simulink model "MPC_WoodBerry_2017a"  (R2017a)
settings: Solver=ode3  SolverName=FixedStepAuto  StartTime=0  StopTime=200  FixedStep=Ts  RelTol=1e-3
values from neighbouring files (symbols this model uses):
  L = Tuning_Parameters.scale.L    [Shell3x3.m]    (also in Shell7x5.m; WoodBerry.m; fpso.m; fpso_tuning.m)
  Ru = Tuning_Parameters.scale.Ru    [Shell3x3.m]    (also in Shell7x5.m; WoodBerry.m; fpso.m; fpso1.m = R(1:ny,1:ny))
  Rv = Tuning_Parameters.scale.Rv    [Shell3x3.m]    (also in Shell7x5.m; WoodBerry.m; fpso.m; fpso1.m = R(ny+1:end,ny+1:end))
libraries: cstblocks x2, mpclib x1
settings Model: Creator=Sergio Castaño  LastModifiedBy=Sergio
settings DataIOCC: LimitDataPoints=on
settings OptimizationCC: DefaultParameterBehavior=Inlined  UseFloatMulNetSlope=on  InlineInvariantSignals=on  EnhancedBackFolding=on  PassReuseOutputArgsAs=Individual arguments  EfficientFloat2IntCast=on  LifeSpan=inf
settings DebuggingCC: ParameterTunabilityLossMsg=error  AllowSymbolicDim=off  SFUnexpectedBacktrackingDiag=warning  SFNoUnconditionalDefaultTransitionDiag=warning  SFExecutionAtInitializationDiag=none
settings HardwareCC: ProdBitPerSizeT=32  ProdBitPerPtrDiffT=32  ProdWordSize=32  ProdHWDeviceType=Specified
settings ModelReferenceCC: UpdateModelReferenceTargets=AssumeUpToDate  CheckModelReferenceTargetMessage=none  EnableParallelModelReferenceBuilds=on  PropagateSignalLabelsOutOfModel=off
settings SFSimCC: MATLABDynamicMemAlloc=off
settings RTWCC: SystemTargetFile=ert.tlc  TemplateMakefile=ert_default_tmf  Description=Embedded Coder  GenerateReport=on  IncludeHyperlinkInReport=on  LaunchReport=on  GenerateTraceInfo=on  GenerateTraceReport=on  GenerateTraceReportSl=on  GenerateTraceReportSf=on  GenerateTraceReportEml=on
settings CodeAppCC: ForceParamTrailComments=on  IgnoreCustomStorageClasses=off  OperatorAnnotations=on  SimulinkDataObjDesc=on  SFDataObjDesc=on  InsertBlockDesc=on
settings ERTTargetCC: GenerateSampleERTMain=on  SupportContinuousTime=on  InlinedParameterPlacement=NonHierarchical  ERTCustomFileTemplate=example_file_process.tlc
settings ConfigComp: CovMetricSettings=dw  CovSaveCumulativeToWorkspaceVar=on  CovSaveSingleToWorkspaceVar=on  CovExternalEMLEnable=off

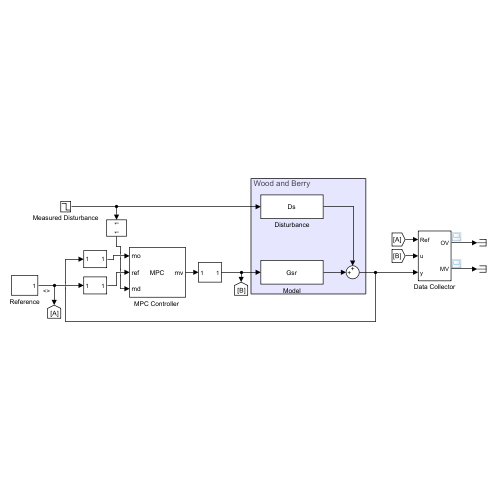
[thumbnail: Simulink's stored preview of the top-level diagram]
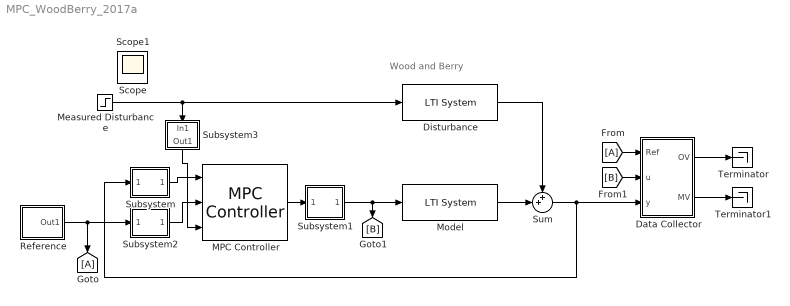
== system MPC_WoodBerry_2017a ==
  note: Wood and Berry
  Data Collector : Subsystem
  Disturbance : cstblocks/LTI System  sys=Ds  IC=[]
  "MPC Controller " : mpclib/MPC Controller  SCDEnableBlockLinearizationSpecification=on  mpcobj=mpc_toolbox  is_multiple=0  enable_value=0  return_u0=off  updateMPCinCallerWorkspace=on  md_inport=on  mv_inport=off  uref_inport=off  cost_outport=off  return_sequence=off  return_qpstatus=off  return_xseq=off  return_state=off  return_ovseq=off  state_inport=off  umin_inport=off  umax_inport=off  ymin_inport=off  ymax_inport=off  cc_inport=off  ywt_inport=off  uwt_inport=off  duwt_inport=off  rhoeps_inport=off  pm_inport=off  MaximumP=10  HorizonChoice=FixedHorizon  n_ts=1  n_p=32  n_mv=2  n_md=1  n_ud=0  n_mo=2  n_uo=0  BlockDataType=double  SampleTimeInherited=off  switch_inport=off
  Measured Disturbance : Step  Time=140  After=-0.25  SampleTime=0
  Model : cstblocks/LTI System  sys=Gsr  IC=[]
  Reference : Subsystem
  Subsystem : Subsystem
  Subsystem1 : Subsystem
  Subsystem2 : Subsystem
  Subsystem3 : Subsystem
  Sum : Sum  Inputs=++|
  Terminator : Terminator
  Terminator1 : Terminator
  Scope : Scope
  Scope1 : Scope
  wires:
  "MPC Controller "/1 -> Subsystem1/1(In1)
  Model/1 -> Sum/2
  Sum/1 -> Data Collector/3(y), Subsystem/1(In1)
  Subsystem/1(Out1) -> "MPC Controller "/1
  Subsystem2/1(Out1) -> "MPC Controller "/2
  Subsystem1/1(Out1) -> [B], Model/1
  Reference/1(Out1) -> [A], Subsystem2/1(In1)
  Measured Disturbance/1 -> Subsystem3/1(In1), Disturbance/1
  [A] -> Data Collector/1(Ref)
  [B] -> Data Collector/2(u)
  Data Collector/1(OV) -> Terminator/1
  Data Collector/2(MV) -> Terminator1/1
  Disturbance/1 -> Sum/1
  Subsystem3/1(Out1) -> "MPC Controller "/3

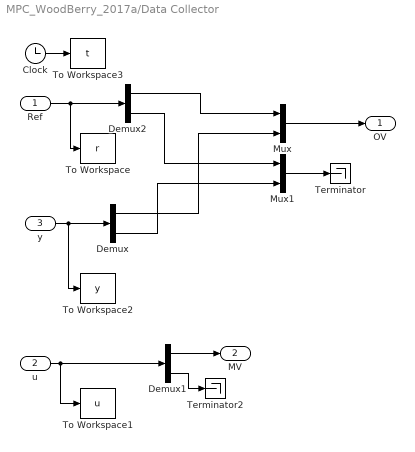
== system MPC_WoodBerry_2017a/Data Collector ==
  Ref : Inport
  u : Inport  Port=2
  y : Inport  Port=3
  Clock : Clock
  Demux : Demux  Outputs=2
  Demux1 : Demux  Outputs=2
  Demux2 : Demux  Outputs=2
  Mux : Mux  Inputs=2
  Mux1 : Mux  Inputs=2
  Terminator : Terminator
  Terminator2 : Terminator
  To Workspace : ToWorkspace  VariableName=r  SampleTime=-1
  To Workspace1 : ToWorkspace  VariableName=u  SampleTime=-1
  To Workspace2 : ToWorkspace  VariableName=y  SampleTime=-1
  To Workspace3 : ToWorkspace  VariableName=t  SampleTime=-1
  OV : Outport
  MV : Outport  Port=2
  wires:
  y/1 -> To Workspace2/1, Demux/1
  u/1 -> Demux1/1, To Workspace1/1
  Ref/1 -> To Workspace/1, Demux2/1
  Demux2/1 -> Mux/1
  Demux/1 -> Mux/2
  Demux2/2 -> Mux1/1
  Demux/2 -> Mux1/2
  Mux/1 -> OV/1
  Mux1/1 -> Terminator/1
  Demux1/1 -> MV/1
  Demux1/2 -> Terminator2/1
  Clock/1 -> To Workspace3/1

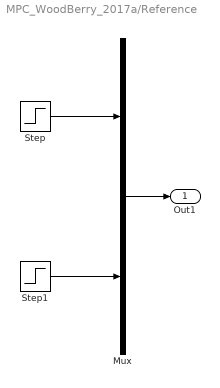
== system MPC_WoodBerry_2017a/Reference ==
  Mux : Mux  Inputs=2
  Step : Step  Time=5  After=0.8  SampleTime=0
  Step1 : Step  Time=60  After=0.5  SampleTime=0
  Out1 : Outport
  wires:
  Mux/1 -> Out1/1
  Step/1 -> Mux/1
  Step1/1 -> Mux/2

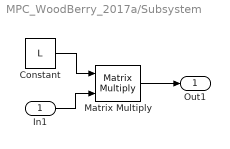
== system MPC_WoodBerry_2017a/Subsystem ==
  In1 : Inport
  Constant : Constant  Value=L
  Matrix Multiply : Product  Multiplication=Matrix(*)
  Out1 : Outport
  wires:
  Matrix Multiply/1 -> Out1/1
  In1/1 -> Matrix Multiply/2
  Constant/1 -> Matrix Multiply/1

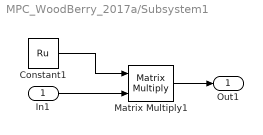
== system MPC_WoodBerry_2017a/Subsystem1 ==
  In1 : Inport
  Constant1 : Constant  Value=Ru
  Matrix Multiply1 : Product  Multiplication=Matrix(*)
  Out1 : Outport
  wires:
  Matrix Multiply1/1 -> Out1/1
  In1/1 -> Matrix Multiply1/2
  Constant1/1 -> Matrix Multiply1/1

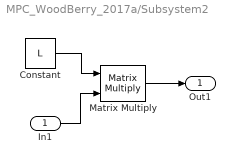
== system MPC_WoodBerry_2017a/Subsystem2 ==
  In1 : Inport
  Constant : Constant  Value=L
  Matrix Multiply : Product  Multiplication=Matrix(*)
  Out1 : Outport
  wires:
  Matrix Multiply/1 -> Out1/1
  Constant/1 -> Matrix Multiply/1
  In1/1 -> Matrix Multiply/2

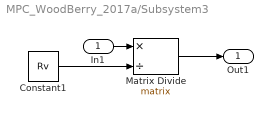
== system MPC_WoodBerry_2017a/Subsystem3 ==
  In1 : Inport
  Constant1 : Constant  Value=Rv
  Matrix Divide : Product  Inputs=*/  Multiplication=Matrix(*)
  Out1 : Outport
  wires:
  Matrix Divide/1 -> Out1/1
  In1/1 -> Matrix Divide/1
  Constant1/1 -> Matrix Divide/2
